simulink model "V1_S_Function_Model"  (R2017a)
settings: Solver=ode45  StartTime=0.0  StopTime=T  MaxStep=0.01  RelTol=1e-3  EnableMultiTasking=on
values from neighbouring files (symbols this model uses):
  g = 9.81    [START.m]    (also in V1_Figure_Data.mat; sFunModell.m = block.DialogPrm(1).Data)
  l1 = 0.2    [START.m]    (also in V1_Figure_Data.mat; sFunModell.m = block.DialogPrm(4).Data)
  l2 = 0.2    [START.m]    (also in V1_Figure_Data.mat; sFunModell.m = block.DialogPrm(5).Data)
  m1 = 0.3    [START.m]    (also in V1_Figure_Data.mat; sFunModell.m = block.DialogPrm(2).Data)
  m2 = 0.3    [START.m]    (also in V1_Figure_Data.mat; sFunModell.m = block.DialogPrm(3).Data)
  Rp1 = 1e-2    (= 0.01)    [START.m]    (also in V1_Figure_Data.mat; sFunModell.m = block.DialogPrm(6).Data)
  Rp2 = 1e-3    (= 0.001)    [START.m]    (also in V1_Figure_Data.mat; sFunModell.m = block.DialogPrm(7).Data)
settings Model: Creator=ajentsch  LastModifiedBy=Ali Kerem Sacakli
settings DataIOCC: LimitDataPoints=on
settings OptimizationCC: LifeSpan=inf
settings DebuggingCC: AllowSymbolicDim=off  SFUnexpectedBacktrackingDiag=warning  SFNoUnconditionalDefaultTransitionDiag=warning  SFExecutionAtInitializationDiag=none
settings ModelReferenceCC: PropagateSignalLabelsOutOfModel=off
settings GRTTargetCC: TargetLangStandard=C89/C90 (ANSI)
settings ConfigComp: CovMetricSettings=dw  CovHtmlReporting=on  CovSaveCumulativeToWorkspaceVar=on  CovSaveSingleToWorkspaceVar=on  CovExternalEMLEnable=off

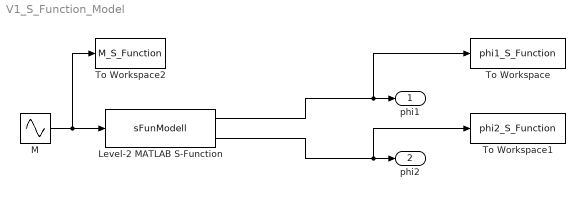
== system V1_S_Function_Model ==
  Level-2 MATLAB S-Function : M-S-Function  FunctionName=sFunModell  Parameters=g,m1,m2,l1,l2,Rp1,Rp2
  M : Sin  Amplitude=0.1  SampleTime=0
  To Workspace : ToWorkspace  VariableName=phi1_S_Function  SaveFormat=Timeseries  SampleTime=-1
  To Workspace1 : ToWorkspace  VariableName=phi2_S_Function  SaveFormat=Timeseries  SampleTime=-1
  To Workspace2 : ToWorkspace  VariableName=M_S_Function  SaveFormat=Timeseries  SampleTime=-1
  phi1 : Outport
  phi2 : Outport  Port=2
  wires:
  M/1 -> To Workspace2/1, Level-2 MATLAB S-Function/1
  Level-2 MATLAB S-Function/1 -> To Workspace/1, phi1/1
  Level-2 MATLAB S-Function/2 -> To Workspace1/1, phi2/1
